simulink model "LKA_ensemble_other"  (R2022a)
settings: Solver=FixedStepAuto  StartTime=0.0  StopTime=T  FixedStep=Ts  RelTol=1e-3
undefined symbols (not defined in the file): actionTable, actionUB, Cf, Cr, DiscIntNeverNeededParam, e1_initial, e2_initial, isAvg, isPred, isTerminate, isVote, Iz, lat_terminate_error, lf, lr, m, max_late_dev, max_rel_yaw_ang, md, rewardToIndex, rewardUB1, rewardUB2, rewardWeights, stateTable, tranTable, Ts, u_max, u_min, Vx
libraries: rllib x9, simulink x1, dspstat3 x1
settings Model: Creator=The MathWorks, Inc.  LastModifiedBy=momentumlab
settings SolverCC: AlgebraicLoopSolver=TrustRegion
settings DataIOCC: ReturnWorkspaceOutputs=off
settings DebuggingCC: UnconnectedInputMsg=warning  UnconnectedOutputMsg=warning  UnconnectedLineMsg=warning  SFMachineParentedDataDiag=warning  ArithmeticOperatorsInVariantConditions=warning
settings SFSimCC: SimUseLocalCustomCode=off  CustomCodeUndefinedFunction=UseInterfaceOnly
settings RTWCC: RTWUseLocalCustomCode=off  DLArmComputeVersion=19.05
settings CodeAppCC: StateflowObjectComments=on
settings SimscapeCC: SimscapeNormalizeSystem=off

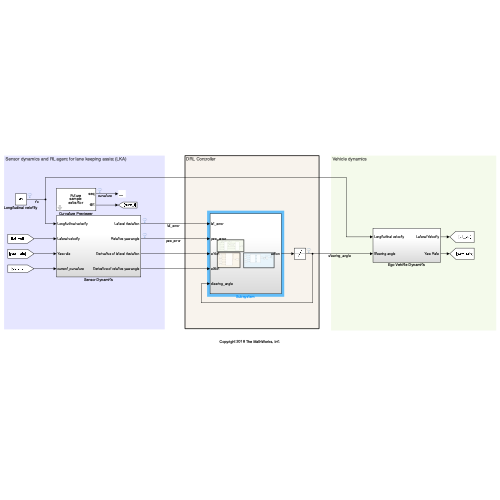
[thumbnail: Simulink's stored preview of the top-level diagram]
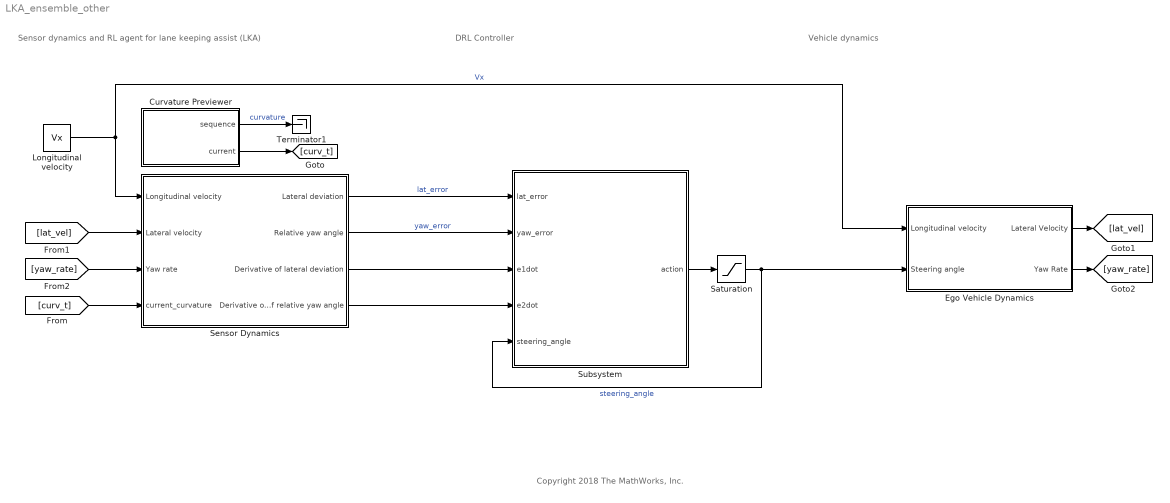
== system LKA_ensemble_other ==
  note: DRL Controller
  note: Vehicle dynamics
  note: Sensor dynamics and RL agent for lane keeping assist (LKA)
  note: Copyright 2018 The MathWorks, Inc.
  Curvature Previewer : Subsystem  mask{signal=md, ts=Ts, steps=10}
      mask prompts: signal "Signal name"; ts "Sampling time"; steps "Number of previewing steps"
      mask init:
      | ts = evalin('base',get_param(gcbh,'ts'));
      | signal = evalin('base',get_param(gcbh,'signal'));
      | steps = evalin('base',get_param(gcbh,'steps'));
      | data = mpc_previewer_maskinit(signal,ts);
      mask Display:
      | fprintf('Future\nsample\nextractor');
      | port_label('output', 1, 'seq')
      | port_label('output', 2, '@t')
  Ego Vehicle Dynamics : Subsystem
  Longitudinal velocity : Constant  Value=Vx  SampleTime=Ts
  Saturation : Saturate  UpperLimit=u_max  LowerLimit=u_min
  Sensor Dynamics : Subsystem
  Subsystem : Subsystem
  Terminator1 : Terminator
  wires:
  Ego Vehicle Dynamics/1(Lateral Velocity) -> [lat_vel]
  Longitudinal velocity/1 -> Ego Vehicle Dynamics/1(Longitudinal velocity), Sensor Dynamics/1(Longitudinal velocity)  "Vx"
  Curvature Previewer/2(current) -> [curv_t]
  [curv_t] -> Sensor Dynamics/4(current_curvature)
  Ego Vehicle Dynamics/2(Yaw Rate) -> [yaw_rate]
  [lat_vel] -> Sensor Dynamics/2(Lateral velocity)
  [yaw_rate] -> Sensor Dynamics/3(Yaw rate)
  Saturation/1 -> Ego Vehicle Dynamics/2(Steering angle), Subsystem/5(steering_angle)  "steering_angle"
  Curvature Previewer/1(sequence) -> Terminator1/1  "curvature"
  Sensor Dynamics/1(Lateral deviation) -> Subsystem/1(lat_error)  "lat_error"
  Sensor Dynamics/2(Relative yaw angle) -> Subsystem/2(yaw_error)  "yaw_error"
  Sensor Dynamics/3(Derivative of lateral deviation) -> Subsystem/3("e1dot ")
  Sensor Dynamics/4(Derivative of relative yaw angle) -> Subsystem/4(e2dot)
  Subsystem/1(action) -> Saturation/1

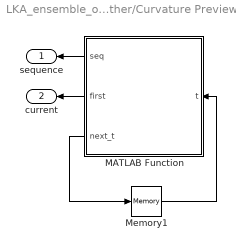
== system LKA_ensemble_other/Curvature Previewer ==
  MATLAB Function : MATLAB Function  TreatAsAtomicUnit=on
  Memory1 : Memory  InheritSampleTime=on  LinearizeAsDelay=on
  sequence : Outport  VectorParamsAs1DForOutWhenUnconnected=off
  current : Outport  Port=2  VectorParamsAs1DForOutWhenUnconnected=off
  wires:
  MATLAB Function/1(seq) -> sequence/1
  MATLAB Function/2(first) -> current/1
  Memory1/1 -> MATLAB Function/1(t)
  MATLAB Function/3(next_t) -> Memory1/1

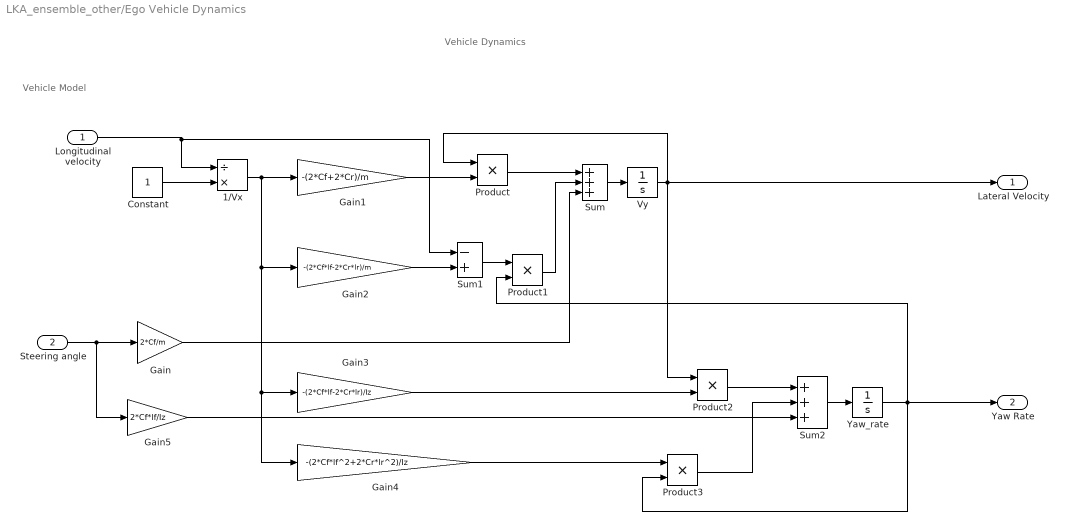
== system LKA_ensemble_other/Ego Vehicle Dynamics ==
  note: Vehicle Model
  note: Vehicle Dynamics
  Longitudinal velocity : Inport
  Steering angle : Inport  Port=2
  1/Vx : Product  Inputs=/*
  Constant : Constant
  Gain : Gain  Gain=2*Cf/m
  Gain1 : Gain  Gain=-(2*Cf+2*Cr)/m
  Gain2 : Gain  Gain=-(2*Cf*lf-2*Cr*lr)/m
  Gain3 : Gain  Gain=-(2*Cf*lf-2*Cr*lr)/Iz
  Gain4 : Gain  Gain=-(2*Cf*lf^2+2*Cr*lr^2)/Iz
  Gain5 : Gain  Gain=2*Cf*lf/Iz
  Product{,1..3} (4 alike) : Product
  Sum : Sum  Inputs=+++
  Sum1 : Sum  Inputs=-+
  Sum2 : Sum  Inputs=+++
  Vy : Integrator
  "Yaw_rate " : Integrator
  Lateral Velocity : Outport  VectorParamsAs1DForOutWhenUnconnected=off
  Yaw Rate : Outport  Port=2  VectorParamsAs1DForOutWhenUnconnected=off
  wires:
  Sum2/1 -> "Yaw_rate "/1
  Gain2/1 -> Sum1/2
  Gain4/1 -> Product3/1
  Constant/1 -> 1/Vx/2
  Gain3/1 -> Product2/2
  1/Vx/1 -> Gain4/1, Gain3/1, Gain2/1, Gain1/1
  Product2/1 -> Sum2/1
  Product3/1 -> Sum2/2
  Gain5/1 -> Sum2/3
  Sum1/1 -> Product1/1
  "Yaw_rate "/1 -> Product3/2, Yaw Rate/1, Product1/2
  Gain/1 -> Sum/3
  Steering angle/1 -> Gain/1, Gain5/1
  Gain1/1 -> Product/2
  Product/1 -> Sum/1
  Vy/1 -> Product/1, Lateral Velocity/1, Product2/1
  Sum/1 -> Vy/1
  Longitudinal velocity/1 -> Sum1/1, 1/Vx/1
  Product1/1 -> Sum/2

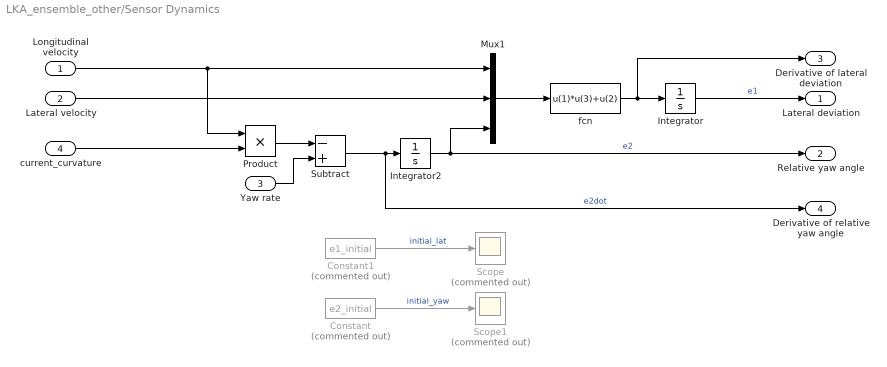
== system LKA_ensemble_other/Sensor Dynamics ==
  Longitudinal velocity : Inport
  Lateral velocity : Inport  Port=2
  Yaw rate : Inport  Port=3
  current_curvature : Inport  Port=4
  Constant : Constant  Commented=on  Value=e2_initial
  Constant1 : Constant  Commented=on  Value=e1_initial
  Integrator : Integrator  InitialCondition=e1_initial
  Integrator2 : Integrator  InitialCondition=e2_initial
  Mux1 : Mux  Inputs=[1 1 1]
  Product : Product
  Scope : Scope  Commented=on
  Scope1 : Scope  Commented=on
  Subtract : Sum  Inputs=-+
  fcn : Fcn  Expr=u(1)*u(3)+u(2)
  Lateral deviation : Outport  VectorParamsAs1DForOutWhenUnconnected=off
  Relative yaw angle : Outport  Port=2  VectorParamsAs1DForOutWhenUnconnected=off
  Derivative of lateral deviation : Outport  Port=3  VectorParamsAs1DForOutWhenUnconnected=off
  Derivative of relative yaw angle : Outport  Port=4  VectorParamsAs1DForOutWhenUnconnected=off
  wires:
  Integrator2/1 -> Relative yaw angle/1, Mux1/3  "e2"
  Mux1/1 -> fcn/1
  fcn/1 -> Derivative of lateral deviation/1, Integrator/1
  Lateral velocity/1 -> Mux1/2
  Integrator/1 -> Lateral deviation/1  "e1"
  Product/1 -> Subtract/1
  Yaw rate/1 -> Subtract/2
  Subtract/1 -> Derivative of relative yaw angle/1, Integrator2/1  "e2dot"
  Longitudinal velocity/1 -> Mux1/1, Product/1
  current_curvature/1 -> Product/2
  Constant1/1 -> Scope/1  "initial_lat"
  Constant/1 -> Scope1/1  "initial_yaw"

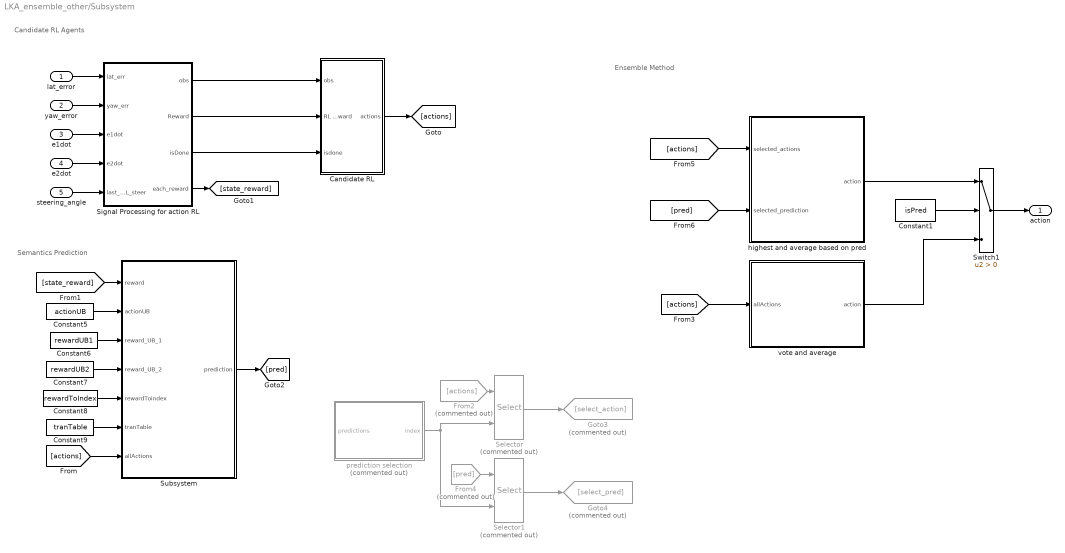
== system LKA_ensemble_other/Subsystem ==
  note: Ensemble Method
  note: Semantics Prediction
  note: Candidate RL Agents
  lat_error : Inport
  yaw_error : Inport  Port=2
  "e1dot " : Inport  Port=3
  e2dot : Inport  Port=4
  steering_angle : Inport  Port=5
  Candidate RL : Subsystem
  Constant1 : Constant  Value=isPred
  Constant5 : Constant  Value=actionUB
  Constant6 : Constant  Value=rewardUB1
  Constant7 : Constant  Value=rewardUB2
  Constant8 : Constant  Value=rewardToIndex
  Constant9 : Constant  Value=tranTable
  From2 : From  Commented=on  GotoTag=actions
  From4 : From  Commented=on  GotoTag=pred
  Goto3 : Goto  Commented=on  GotoTag=select_action
  Goto4 : Goto  Commented=on  GotoTag=select_pred
  Selector : Selector  Commented=on  InputPortWidth=3  IndexOptions=Index vector (port)  Indices=[1 3]  OutputSizes=1
  Selector1 : Selector  Commented=on  InputPortWidth=3  IndexOptions=Index vector (port)  Indices=[1 3]  OutputSizes=1
  "Signal Processing for action RL " : Subsystem
  Subsystem : Subsystem
  Switch1 : Switch  Criteria=u2 > Threshold  SaturateOnIntegerOverflow=off  InputSameDT=off
  highest and average based on pred : Subsystem
  prediction selection : MATLAB Function  Commented=on  TreatAsAtomicUnit=on
  vote and average : Subsystem
  action : Outport
  wires:
  yaw_error/1 -> "Signal Processing for action RL "/2(yaw_err)
  e2dot/1 -> "Signal Processing for action RL "/4(e2dot)
  steering_angle/1 -> "Signal Processing for action RL "/5(last_RL_steer)
  "e1dot "/1 -> "Signal Processing for action RL "/3("e1dot ")
  lat_error/1 -> "Signal Processing for action RL "/1(lat_err)
  "Signal Processing for action RL "/1(obs) -> Candidate RL/1(obs)
  "Signal Processing for action RL "/2(Reward) -> Candidate RL/2(RL reward)
  "Signal Processing for action RL "/3(isDone) -> Candidate RL/3(isdone)
  Candidate RL/1(actions) -> [actions]
  Subsystem/1(prediction) -> [pred]
  prediction selection/1(index) -> Selector/2, Selector1/2
  From2/1 -> Selector/1
  [actions] -> vote and average/1(allActions)
  Selector/1 -> Goto3/1
  From4/1 -> Selector1/1
  Constant1/1 -> Switch1/2
  Switch1/1 -> action/1
  vote and average/1(action) -> Switch1/3
  highest and average based on pred/1(action) -> Switch1/1
  Selector1/1 -> Goto4/1
  [actions] -> highest and average based on pred/1(selected_actions)
  [pred] -> highest and average based on pred/2(selected_prediction)
  Constant5/1 -> Subsystem/2(actionUB)
  Constant9/1 -> Subsystem/6(tranTable)
  Constant6/1 -> Subsystem/3(reward_UB_1)
  Constant7/1 -> Subsystem/4(reward_UB_2)
  Constant8/1 -> Subsystem/5(rewardToindex)
  [actions] -> Subsystem/7(allActions)
  [state_reward] -> Subsystem/1(reward)
  "Signal Processing for action RL "/4(each_reward) -> [state_reward]

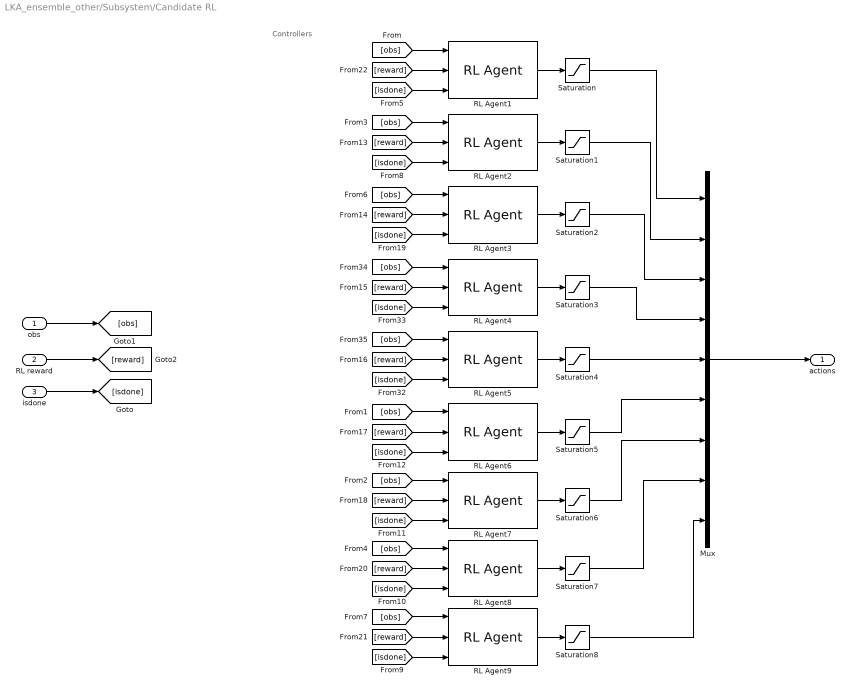
== system LKA_ensemble_other/Subsystem/Candidate RL ==
  note: Controllers
  obs : Inport
  RL reward : Inport  Port=2
  isdone : Inport  Port=3
  Mux : Mux  Inputs=9
  RL Agent1 : rllib/RL Agent  Agent=agent1  ExternalActionAsInput=off  ProvideLastAction=off  ProvideCumRwd=off  TreatAsDirectFeedthrough=on  UseStrictObservationDataTypes=off
  RL Agent2 : rllib/RL Agent  Agent=agent2  ExternalActionAsInput=off  ProvideLastAction=off  ProvideCumRwd=off  TreatAsDirectFeedthrough=on  UseStrictObservationDataTypes=off
  RL Agent3 : rllib/RL Agent  Agent=agent3  ExternalActionAsInput=off  ProvideLastAction=off  ProvideCumRwd=off  TreatAsDirectFeedthrough=on  UseStrictObservationDataTypes=off
  RL Agent4 : rllib/RL Agent  Agent=agent3  ExternalActionAsInput=off  ProvideLastAction=off  ProvideCumRwd=off  TreatAsDirectFeedthrough=on  UseStrictObservationDataTypes=off
  RL Agent5 : rllib/RL Agent  Agent=agent3  ExternalActionAsInput=off  ProvideLastAction=off  ProvideCumRwd=off  TreatAsDirectFeedthrough=on  UseStrictObservationDataTypes=off
  RL Agent6 : rllib/RL Agent  Agent=agent6  ExternalActionAsInput=off  ProvideLastAction=off  ProvideCumRwd=off  TreatAsDirectFeedthrough=on  UseStrictObservationDataTypes=off
  RL Agent7 : rllib/RL Agent  Agent=agent7  ExternalActionAsInput=off  ProvideLastAction=off  ProvideCumRwd=off  TreatAsDirectFeedthrough=on  UseStrictObservationDataTypes=off
  RL Agent8 : rllib/RL Agent  Agent=agent8  ExternalActionAsInput=off  ProvideLastAction=off  ProvideCumRwd=off  TreatAsDirectFeedthrough=on  UseStrictObservationDataTypes=off
  RL Agent9 : rllib/RL Agent  Agent=agent9  ExternalActionAsInput=off  ProvideLastAction=off  ProvideCumRwd=off  TreatAsDirectFeedthrough=on  UseStrictObservationDataTypes=off
  Saturation{,1..8} (9 alike) : Saturate  UpperLimit=u_max  LowerLimit=u_min
  actions : Outport
  wires:
  [obs] -> RL Agent7/1
  [obs] -> RL Agent4/1
  [obs] -> RL Agent3/1
  Saturation3/1 -> Mux/4
  [obs] -> RL Agent1/1
  [isdone] -> RL Agent1/3
  [obs] -> RL Agent2/1
  [obs] -> RL Agent5/1
  RL Agent1/1 -> Saturation/1
  [isdone] -> RL Agent8/3
  [isdone] -> RL Agent6/3
  RL reward/1 -> [reward]
  Saturation/1 -> Mux/1
  RL Agent6/1 -> Saturation5/1
  Saturation4/1 -> Mux/5
  RL Agent3/1 -> Saturation2/1
  [isdone] -> RL Agent2/3
  [isdone] -> RL Agent7/3
  RL Agent8/1 -> Saturation7/1
  Saturation1/1 -> Mux/2
  [isdone] -> RL Agent5/3
  Mux/1 -> actions/1
  [obs] -> RL Agent6/1
  [isdone] -> RL Agent3/3
  RL Agent5/1 -> Saturation4/1
  RL Agent4/1 -> Saturation3/1
  RL Agent7/1 -> Saturation6/1
  RL Agent2/1 -> Saturation1/1
  [obs] -> RL Agent8/1
  Saturation2/1 -> Mux/3
  [isdone] -> RL Agent4/3
  RL Agent9/1 -> Saturation8/1
  [obs] -> RL Agent9/1
  [isdone] -> RL Agent9/3
  Saturation5/1 -> Mux/6
  Saturation6/1 -> Mux/7
  Saturation7/1 -> Mux/8
  Saturation8/1 -> Mux/9
  isdone/1 -> [isdone]
  obs/1 -> [obs]
  [reward] -> RL Agent2/2
  [reward] -> RL Agent3/2
  [reward] -> RL Agent4/2
  [reward] -> RL Agent5/2
  [reward] -> RL Agent6/2
  [reward] -> RL Agent7/2
  [reward] -> RL Agent8/2
  [reward] -> RL Agent9/2
  [reward] -> RL Agent1/2

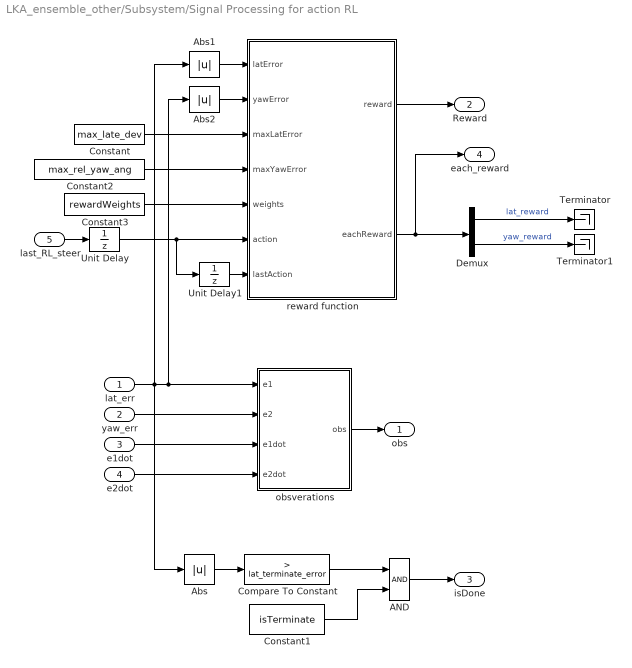
== system LKA_ensemble_other/Subsystem/Signal Processing for action RL  ==
  lat_err : Inport
  yaw_err : Inport  Port=2
  "e1dot " : Inport  Port=3
  e2dot : Inport  Port=4
  last_RL_steer : Inport  Port=5
  AND : Logic  IconShape=distinctive  AllPortsSameDT=off  OutDataTypeStr=boolean
  Abs : Abs  SaturateOnIntegerOverflow=off
  Abs1 : Abs  SaturateOnIntegerOverflow=off
  Abs2 : Abs  SaturateOnIntegerOverflow=off
  Compare To Constant : simulink/Logic and Bit Operations/Compare To Constant  relop=>  const=lat_terminate_error  OutDataTypeStr=boolean
  Constant : Constant  Value=max_late_dev
  Constant1 : Constant  Value=isTerminate
  Constant2 : Constant  Value=max_rel_yaw_ang
  Constant3 : Constant  Value=rewardWeights
  Demux : Demux  Outputs=2
  Terminator : Terminator
  Terminator1 : Terminator
  Unit Delay : UnitDelay  SampleTime=-1  HasFrameUpgradeWarning=on
  Unit Delay1 : UnitDelay  SampleTime=-1  HasFrameUpgradeWarning=on
  obsverations : Subsystem
  reward function : MATLAB Function  TreatAsAtomicUnit=on
  obs : Outport  VectorParamsAs1DForOutWhenUnconnected=off
  Reward : Outport  Port=2  VectorParamsAs1DForOutWhenUnconnected=off
  isDone : Outport  Port=3  VectorParamsAs1DForOutWhenUnconnected=off
  each_reward : Outport  Port=4
  wires:
  obsverations/1(obs) -> obs/1
  "e1dot "/1 -> obsverations/3(e1dot)
  e2dot/1 -> obsverations/4(e2dot)
  yaw_err/1 -> obsverations/2(e2)
  lat_err/1 -> obsverations/1(e1), Abs2/1, Abs1/1, Abs/1
  reward function/1(reward) -> Reward/1
  Constant/1 -> reward function/3(maxLatError)
  Abs1/1 -> reward function/1(latError)
  Abs2/1 -> reward function/2(yawError)
  last_RL_steer/1 -> Unit Delay/1
  Abs/1 -> Compare To Constant/1
  Compare To Constant/1 -> AND/1
  Constant1/1 -> AND/2
  AND/1 -> isDone/1
  Constant3/1 -> reward function/5(weights)
  Unit Delay1/1 -> reward function/7(lastAction)
  Constant2/1 -> reward function/4(maxYawError)
  Unit Delay/1 -> Unit Delay1/1, reward function/6(action)
  reward function/2(eachReward) -> each_reward/1, Demux/1
  Demux/1 -> Terminator/1  "lat_reward"
  Demux/2 -> Terminator1/1  "yaw_reward"

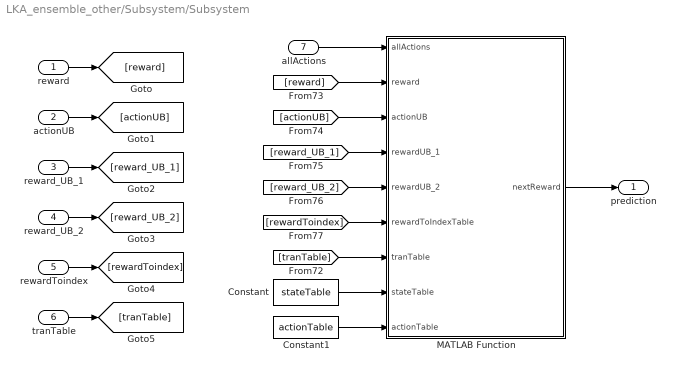
== system LKA_ensemble_other/Subsystem/Subsystem ==
  reward : Inport
  actionUB : Inport  Port=2
  reward_UB_1 : Inport  Port=3
  reward_UB_2 : Inport  Port=4
  rewardToindex : Inport  Port=5
  tranTable : Inport  Port=6
  allActions : Inport  Port=7
  Constant : Constant  Value=stateTable
  Constant1 : Constant  Value=actionTable
  MATLAB Function : MATLAB Function  TreatAsAtomicUnit=on
  prediction : Outport
  wires:
  reward/1 -> [reward]
  rewardToindex/1 -> [rewardToindex]
  actionUB/1 -> [actionUB]
  reward_UB_1/1 -> [reward_UB_1]
  reward_UB_2/1 -> [reward_UB_2]
  tranTable/1 -> [tranTable]
  MATLAB Function/1(nextReward) -> prediction/1
  Constant/1 -> MATLAB Function/8(stateTable)
  allActions/1 -> MATLAB Function/1(allActions)
  [reward_UB_2] -> MATLAB Function/5(rewardUB_2)
  Constant1/1 -> MATLAB Function/9(actionTable)
  [rewardToindex] -> MATLAB Function/6(rewardToIndexTable)
  [reward] -> MATLAB Function/2(reward)
  [tranTable] -> MATLAB Function/7(tranTable)
  [actionUB] -> MATLAB Function/3(actionUB)
  [reward_UB_1] -> MATLAB Function/4(rewardUB_1)

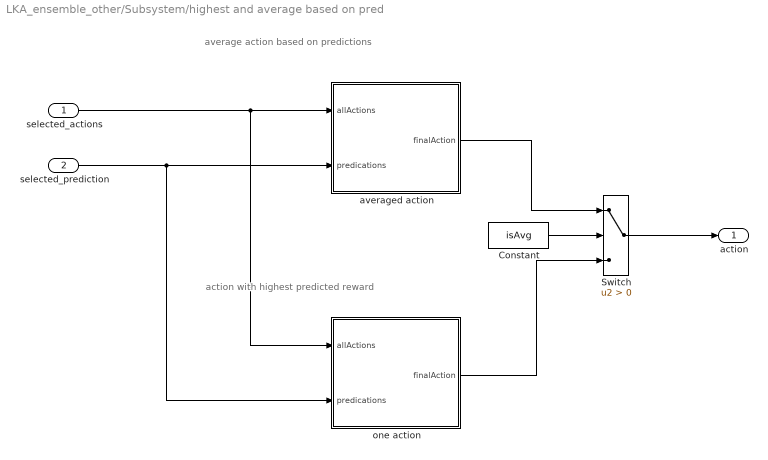
== system LKA_ensemble_other/Subsystem/highest and average based on pred ==
  note: action with highest predicted reward
  note: average action based on predictions
  selected_actions : Inport
  selected_prediction : Inport  Port=2
  Constant : Constant  Value=isAvg
  Switch : Switch  Criteria=u2 > Threshold  SaturateOnIntegerOverflow=off  InputSameDT=off
  averaged action : MATLAB Function  TreatAsAtomicUnit=on
  one action : MATLAB Function  TreatAsAtomicUnit=on
  action : Outport
  wires:
  selected_actions/1 -> averaged action/1(allActions), one action/1(allActions)
  selected_prediction/1 -> one action/2(predications), averaged action/2(predications)
  one action/1(finalAction) -> Switch/3
  Switch/1 -> action/1
  Constant/1 -> Switch/2
  averaged action/1(finalAction) -> Switch/1

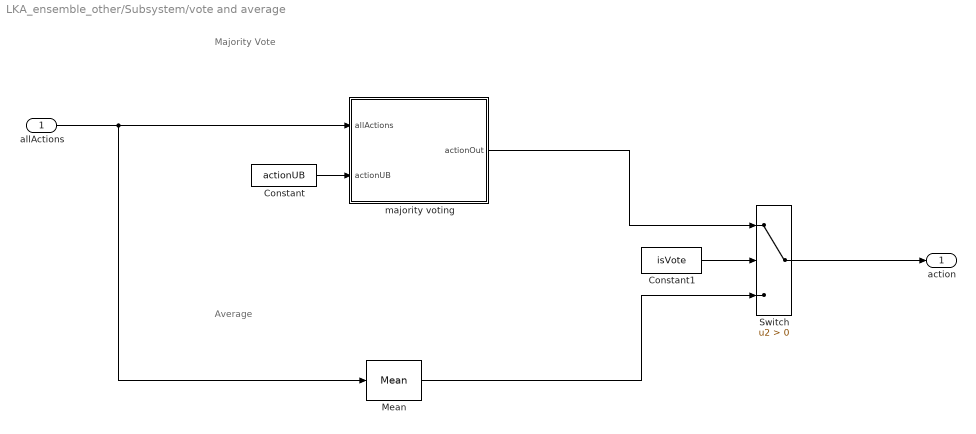
== system LKA_ensemble_other/Subsystem/vote and average ==
  note: Majority Vote
  note: Average
  allActions : Inport
  Constant : Constant  Value=actionUB
  Constant1 : Constant  Value=isVote
  Mean : dspstat3/Mean  run=off  InputProcessing=Columns as channels (frame based)  reset_popup=None  directionMode=Entire input  dimension=1  roiEnable=off  roiType=Rectangles  roiPortion=Entire ROI  roiOutput=Individual statistics for each ROI  roiFlag=off  roundingMode=Floor  overflowMode=off  outputDataTypeStr=Inherit: Same as accumulator  outputMin=[]  outputMax=[]  outputLastDataTypeStr=Inherit: Same as accumulator
  Switch : Switch  Criteria=u2 > Threshold  SaturateOnIntegerOverflow=off  InputSameDT=off
  majority voting : MATLAB Function  TreatAsAtomicUnit=on
  action : Outport
  wires:
  allActions/1 -> Mean/1, majority voting/1(allActions)
  Switch/1 -> action/1
  Constant/1 -> majority voting/2(actionUB)
  majority voting/1(actionOut) -> Switch/1
  Mean/1 -> Switch/3
  Constant1/1 -> Switch/2

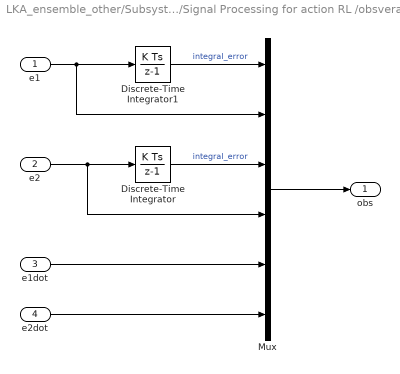
== system LKA_ensemble_other/Subsystem/Signal Processing for action RL /obsverations ==
  e1 : Inport
  e2 : Inport  Port=2
  e1dot : Inport  Port=3
  e2dot : Inport  Port=4
  Discrete-Time Integrator : DiscreteIntegrator  SampleTime=-1  ICPrevOutput=DiscIntNeverNeededParam  ICPrevScaledInput=DiscIntNeverNeededParam
  Discrete-Time Integrator1 : DiscreteIntegrator  SampleTime=-1  ICPrevOutput=DiscIntNeverNeededParam  ICPrevScaledInput=DiscIntNeverNeededParam
  Mux : Mux  Inputs=6
  obs : Outport  VectorParamsAs1DForOutWhenUnconnected=off
  wires:
  e1/1 -> Mux/2, Discrete-Time Integrator1/1
  Mux/1 -> obs/1
  Discrete-Time Integrator1/1 -> Mux/1  "integral_error"
  e2/1 -> Mux/4, Discrete-Time Integrator/1
  Discrete-Time Integrator/1 -> Mux/3  "integral_error"
  e1dot/1 -> Mux/5
  e2dot/1 -> Mux/6

== matlab function LKA_ensemble_other/Subsystem/Signal Processing for action RL /reward function ==
  data: latError input; reward output; yawError input; maxLatError input; maxYawError input; weights input; action input; lastAction input; eachReward output
function [reward,eachReward] = fcn(latError, yawError, maxLatError, maxYawError, weights, action, lastAction)


if latError <= maxLatError
    latReward = tanh(3*abs(maxLatError-latError));
else
    latReward = -tanh(3*abs(maxLatError-latError));
end


if yawError <= maxYawError
    yawReward = tanh(8*abs(maxYawError-yawError));
else
    yawReward = -tanh(9*abs(maxYawError-yawError));
end

stepReward = 0.05;
stableReward = -(action-lastAction)^2;

reward = weights(1)*latReward + weights(2)*yawReward + weights(3)*stableReward + stepReward;
eachReward = [latReward,yawReward];

== matlab function LKA_ensemble_other/Curvature Previewer/MATLAB Function ==
  settings: updateMethod=DISCRETE  sampleTime=ts
  data: data parameter; seq output; steps parameter; t input; first output; next_t output
function [seq,first,next_t] = fcn(data,steps,t)
%#codegen
[seq,first,next_t] = mpcblock_preview('md',data,steps,t);

== matlab function LKA_ensemble_other/Subsystem/Subsystem/MATLAB Function ==
  data: allActions input; nextReward output; reward input; actionUB input; rewardUB_1 input; rewardUB_2 input; rewardToIndexTable input; tranTable input; stateTable input; actionTable input
function nextReward  = fcn(allActions, reward, actionUB, rewardUB_1,rewardUB_2, rewardToIndexTable, tranTable, stateTable,actionTable)

numController = 9;

nextReward = ones(numController, 1);
abReward_1 = find(rewardUB_1 >= reward(1), 1, 'first');  % concrete state -> abstract state
abReward_2 = find(rewardUB_2 >= reward(2), 1, 'first');

if isempty(abReward_1) || isempty(abReward_2)      % if this is an unseen reward
    nextReward = zeros(numController,1);
else
    rewardIndex1 = rewardToIndexTable(:,1)==abReward_1;
    rewardIndex2 = rewardToIndexTable(:,2)==abReward_2;
    
    if isempty(rewardIndex1) || isempty(rewardIndex2)      % if this is an unseen abstract state
        nextReward = zeros(numController,1);
    else
        abState = rewardToIndexTable(rewardToIndexTable(:,1)==abReward_1 & rewardToIndexTable(:,2)==abReward_2, 3);
        
        if isempty(abState)
            nextReward = zeros(numController,1);
        else
            for i = 1:numController
            
                action = allActions(i);
                abAction = find(actionUB >= action, 1, 'first');      % concrete action -> abstract action
            
                stateIndex = stateTable==abState;
                actionindex = actionTable==abAction;
            
                if isempty(stateIndex) || isempty(actionindex)  % if this is an unseen abstract state-action pair
                    abTranReward = 0;
                else
                    temp = stateIndex + actionindex;
                    if ismember(2,temp)
                        abTranReward = tranTable((stateIndex & actionindex),5);
                    else
                        abTranReward = 0;
                    end
                end
                nextReward(i,1) = abTranReward;
            end
        end
    end
end

== matlab function LKA_ensemble_other/Subsystem/prediction selection ==
  data: predictions input; index output
function index = fcn(predictions)

actions = reshape(predictions,[3,9]);
actions = actions';

% only take actions with non-negative predicitons 
index = actions(:,1)>=0 & actions(:,2)>=0;

if sum(index) == 0
    index = 1:9;
else
    index = nonzeros(index.*(1:5))';
    
end

== matlab function LKA_ensemble_other/Subsystem/vote and average/majority voting ==
  data: actionOut output; allActions input; actionUB input
function actionOut = fcn(allActions, actionUB)

numController = 9;

abstractAction = zeros(numController, 2);

for i = 1:numController
    abstractAction(i,1) = find(actionUB >= allActions(i), 1, 'first');      % concrete action -> abstract action;
    abstractAction(i,2) = allActions(i);
end

[GC,GR] = groupcounts(abstractAction(:,1));
actionIndex = GR(GC==max(GC));
actionIndex = ismember(abstractAction(:,1),actionIndex);
actionOut = mean(abstractAction(actionIndex,2));

== matlab function LKA_ensemble_other/Subsystem/highest and average based on pred/averaged action ==
  data: allActions input; finalAction output; predications input
function finalAction = fcn(allActions, predications)

% average of actions with top 3 highest predicted rewards

selectPred = predications(predications>=0);

if isempty(selectPred)
    actionPred = cat(2, allActions,predications);
    actionPred = sortrows(actionPred,2,'descend');
    finalAction = mean(actionPred(1:3,1));
else
    selectAction = allActions(predications>=0);
    actionPred = cat(2, selectAction,selectPred);
    actionPred = sortrows(actionPred,2,'descend');
    if length(actionPred) <3
        finalAction = mean(actionPred(:,1));
    else
        finalAction = mean(actionPred(1:3,1));
    end

end

== matlab function LKA_ensemble_other/Subsystem/highest and average based on pred/one action ==
  data: allActions input; finalAction output; predications input
function finalAction = fcn(allActions, predications)

% take the action with highest predicted reward
[~, idx] = max(predications);
finalAction = allActions(idx);
